simulink model "F18_Sim_animateFG4"  (R2014a)
settings: Solver=ode45  StartTime=0.0  StopTime=sim_time  RelTol=1e-3
values from neighbouring files (symbols this model uses):
  enableRT = 1    [F18_Animation_run3.m]    (also in f18full_DUopenloop_run1.m)
  h_ref = 0    [F18_Animation_run3.m]
  speedRT = 1    [F18_Animation_run3.m]
undefined symbols (not defined in the file or in its folder): Earth, WGS84
libraries: aerolibfltsims x4, aerolibanimutils x1, aerolibtransform2 x1
settings Model: Creator=Mishah  LastModifiedBy=changbc
settings DataIOCC: ExternalInput=[t, y, u]  LimitDataPoints=off  LoadExternalInput=on  SaveOutput=off  SignalLogging=off  SaveTime=off
settings OptimizationCC: ExpressionDepthLimit=2147483647
settings DebuggingCC: UnderspecifiedInitializationDetection=Classic  StateNameClashWarn=warning
settings GRTTargetCC: CombineOutputUpdateFcns=off  GRTInterface=on

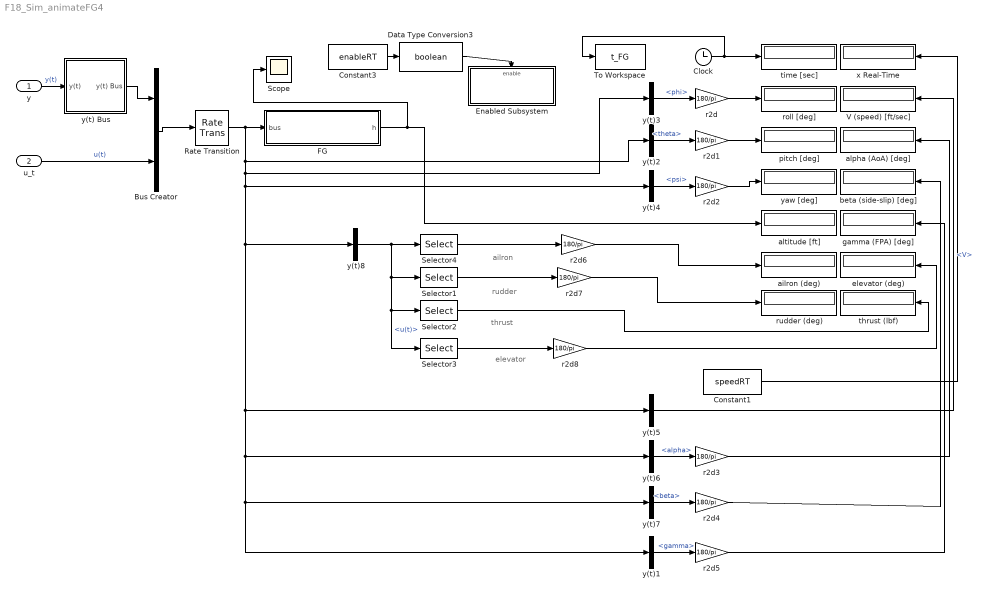
== system F18_Sim_animateFG4 ==
  note: ailron
  note: rudder
  note: thrust
  note: elevator
  y : Inport
  u_t : Inport  Port=2
  Bus Creator : BusCreator  Inputs=2
  Clock : Clock
  Constant1 : Constant  Value=speedRT
  Constant3 : Constant  Value=enableRT
  Data Type Conversion3 : DataTypeConversion  OutDataTypeStr=boolean
  Enabled Subsystem : Subsystem  TreatAsAtomicUnit=on
  FG : Subsystem
  Rate Transition : RateTransition
  Scope : Scope
      settings: YMin=-1000  YMax=12000
  Selector1 : Selector  InputPortWidth=4  Indices=2
  Selector2 : Selector  InputPortWidth=4  Indices=4
  Selector3 : Selector  InputPortWidth=4  Indices=3
  Selector4 : Selector  InputPortWidth=4
  To Workspace : ToWorkspace  VariableName=t_FG  SaveFormat=Structure  SampleTime=-1
  V (speed) [ft/sec] : Display
      settings: Format=bank
  ailron (deg) : Display
      settings: Format=bank
  alpha (AoA) [deg] : Display
      settings: Format=bank
  altitude [ft] : Display
      settings: Format=bank
  beta (side-slip) [deg] : Display
      settings: Format=bank
  elevator (deg) : Display
      settings: Format=bank
  gamma (FPA) [deg] : Display
      settings: Format=bank
  pitch [deg] : Display
      settings: Format=bank
  r2d{,1..8} (9 alike) : Gain  Gain=180/pi
  roll [deg] : Display
      settings: Format=bank
  rudder (deg) : Display
      settings: Format=bank
  thrust (lbf) : Display
      settings: Format=bank
  time [sec] : Display
      settings: Format=bank
  x Real-Time : Display
      settings: Format=bank
  y(t) Bus : Subsystem
  y(t)1 : BusSelector  OutputSignals=y(t) bus.uvwg.gamma
  y(t)2 : BusSelector  OutputSignals=y(t) bus.euler.theta
  y(t)3 : BusSelector  OutputSignals=y(t) bus.euler.phi
  y(t)4 : BusSelector  OutputSignals=y(t) bus.euler.psi
  y(t)5 : BusSelector  OutputSignals=y(t) bus.V;beta;alpha.V
  y(t)6 : BusSelector  OutputSignals=y(t) bus.V;beta;alpha.alpha
  y(t)7 : BusSelector  OutputSignals=y(t) bus.V;beta;alpha.beta
  y(t)8 : BusSelector  OutputSignals=u(t)
  yaw [deg] : Display
      settings: Format=bank
  wires:
  Constant3/1 -> Data Type Conversion3/1
  Rate Transition/1 -> y(t)7/1, y(t)1/1, y(t)6/1, y(t)5/1, y(t)8/1, y(t)4/1, y(t)3/1, y(t)2/1, FG/1(bus)
  y(t) Bus/1(y(t) Bus) -> Bus Creator/1
  u_t/1 -> Bus Creator/2  "u(t)"
  Clock/1 -> time [sec]/1, To Workspace/1
  Bus Creator/1 -> Rate Transition/1
  y(t)3/1 -> r2d/1  "<phi>"
  r2d/1 -> roll [deg]/1
  y(t)2/1 -> r2d1/1  "<theta>"
  r2d1/1 -> pitch [deg]/1
  y(t)4/1 -> r2d2/1  "<psi>"
  r2d2/1 -> yaw [deg]/1
  y(t)5/1 -> V (speed) [ft/sec]/1  "<V>"
  y(t)6/1 -> r2d3/1  "<alpha>"
  r2d3/1 -> alpha (AoA) [deg]/1
  y(t)7/1 -> r2d4/1  "<beta>"
  r2d4/1 -> beta (side-slip) [deg]/1
  y(t)1/1 -> r2d5/1  "<gamma>"
  r2d5/1 -> gamma (FPA) [deg]/1
  Data Type Conversion3/1 -> Enabled Subsystem/Enable
  Constant1/1 -> x Real-Time/1
  y/1 -> y(t) Bus/1(y(t))  "y(t)"
  FG/1(h) -> altitude [ft]/1, Scope/1
  y(t)8/1 -> Selector4/1, Selector1/1, Selector2/1, Selector3/1  "<u(t)>"
  Selector4/1 -> r2d6/1
  Selector1/1 -> r2d7/1
  Selector2/1 -> thrust (lbf)/1
  Selector3/1 -> r2d8/1
  r2d6/1 -> ailron (deg)/1
  r2d7/1 -> rudder (deg)/1
  r2d8/1 -> elevator (deg)/1

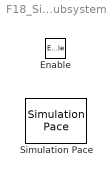
== system F18_Sim_animateFG4/Enabled Subsystem ==
  Enable : EnablePort
  Simulation Pace : aerolibanimutils/Simulation Pace  SimulationPace=1  SleepMode=MATLAB Thread  OutputPaceError=off  SampleTime=1/100
      settings: AttributesFormatString=%<SimulationPace> sec/sec

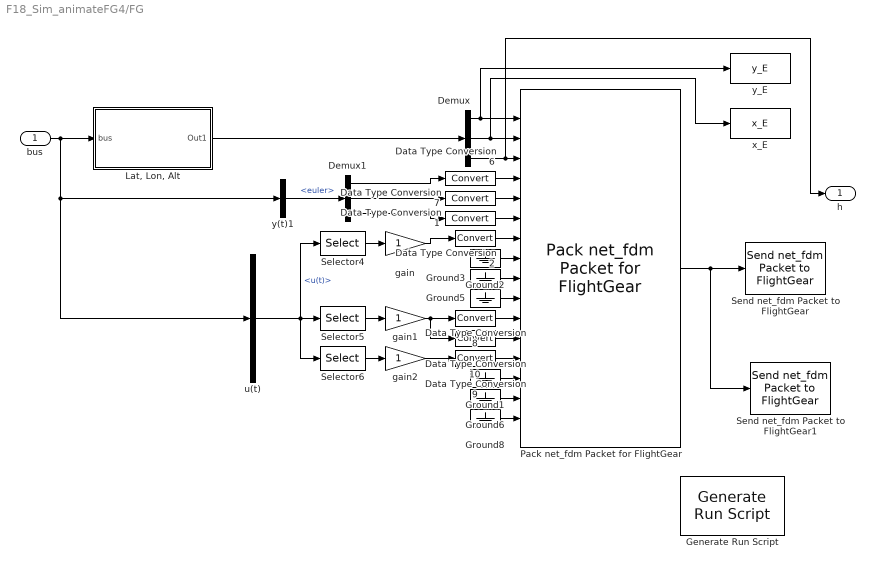
== system F18_Sim_animateFG4/FG ==
  bus : Inport
  Data Type Conversion{1..2,6..10} (7 alike) : DataTypeConversion
  Demux : Demux  Outputs=3
  Demux1 : Demux  Outputs=3
  Generate Run Script : aerolibfltsims/Generate Run Script  OutputFileName=runfg.bat  FlightGearBaseDirectory=C:\Program Files\FlightGear  GeometryModelName=ufo  DestinationPort=5502  OriginAddress=127.0.0.1  OriginPort=5505  LocalAddress=127.0.0.1  AirportId=REMOVE_THIS_LINE_FROM_SCRIPT  RunwayId=10L  InitialAltitude=100  InitialHeading=0  OffsetDistance=0  OffsetAzimuth=0  GenerateFile=off  Architecture=Default  dataFlow=Send
  Ground{1..3,5..6,8} (6 alike) : Ground
  "Lat, Lon, Alt" : Subsystem
  Pack net_fdm Packet for FlightGear : aerolibfltsims/Pack net_fdm Packet for FlightGear  FlightGearVersion=v2.12  ShowPositionAttitudeInputs=on  ShowVelocityAccelerationInputs=off  ShowControlSurfacePositionInputs=on  ShowEngineFuelInputs=off  ShowLandingGearInputs=off  ShowEnvironmentInputs=off  SampleTime=-1
  Selector4 : Selector  InputPortWidth=4  Indices=2
  Selector5 : Selector  InputPortWidth=4  Indices=3
  Selector6 : Selector  InputPortWidth=4  Indices=4
  Send net_fdm Packet to FlightGear : aerolibfltsims/Send net_fdm Packet to FlightGear  DestinationIpAddress=127.0.0.1  DestinationPort=5502  LocalIpPort=-1  varLen=off  SampleTime=-1
  Send net_fdm Packet to FlightGear1 : aerolibfltsims/Send net_fdm Packet to FlightGear  DestinationIpAddress=127.0.0.1  DestinationPort=5602  LocalIpPort=-1  varLen=off  SampleTime=-1
  gain : Gain
  gain1 : Gain
  gain2 : Gain
  u(t) : BusSelector  OutputSignals=u(t)
  x_E : ToWorkspace  VariableName=x_E  SaveFormat=Structure  SampleTime=-1
  y(t)1 : BusSelector  OutputSignals=y(t) bus.euler
  y_E : ToWorkspace  VariableName=y_E  SaveFormat=Structure  SampleTime=-1
  h : Outport
  wires:
  Ground2/1 -> Pack net_fdm Packet for FlightGear/8
  Ground8/1 -> Pack net_fdm Packet for FlightGear/16
  Ground6/1 -> Pack net_fdm Packet for FlightGear/15
  Data Type Conversion9/1 -> Pack net_fdm Packet for FlightGear/13
  Data Type Conversion10/1 -> Pack net_fdm Packet for FlightGear/12
  Data Type Conversion8/1 -> Pack net_fdm Packet for FlightGear/11
  Ground5/1 -> Pack net_fdm Packet for FlightGear/10
  Ground3/1 -> Pack net_fdm Packet for FlightGear/9
  y(t)1/1 -> Demux1/1  "<euler>"
  Data Type Conversion2/1 -> Pack net_fdm Packet for FlightGear/7
  Data Type Conversion1/1 -> Pack net_fdm Packet for FlightGear/6
  Data Type Conversion7/1 -> Pack net_fdm Packet for FlightGear/5
  Data Type Conversion6/1 -> Pack net_fdm Packet for FlightGear/4
  Ground1/1 -> Pack net_fdm Packet for FlightGear/14
  Demux1/3 -> Data Type Conversion1/1
  Demux1/2 -> Data Type Conversion7/1
  Demux1/1 -> Data Type Conversion6/1
  Demux/3 -> Pack net_fdm Packet for FlightGear/3, h/1
  Demux/2 -> Pack net_fdm Packet for FlightGear/2, x_E/1
  Demux/1 -> Pack net_fdm Packet for FlightGear/1, y_E/1
  Pack net_fdm Packet for FlightGear/1 -> Send net_fdm Packet to FlightGear1/1, Send net_fdm Packet to FlightGear/1
  "Lat, Lon, Alt"/1(Out1) -> Demux/1
  u(t)/1 -> Selector4/1, Selector5/1, Selector6/1  "<u(t)>"
  Selector4/1 -> gain/1
  Selector5/1 -> gain1/1
  Selector6/1 -> gain2/1
  gain1/1 -> Data Type Conversion8/1, Data Type Conversion10/1
  gain2/1 -> Data Type Conversion9/1
  gain/1 -> Data Type Conversion2/1
  bus/1 -> u(t)/1, y(t)1/1, "Lat, Lon, Alt"/1(bus)

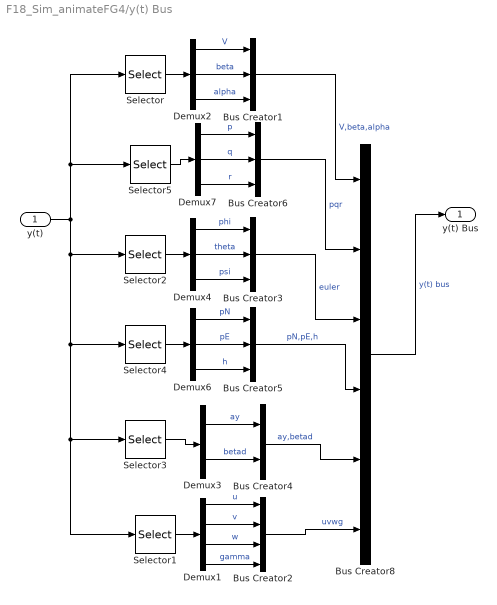
== system F18_Sim_animateFG4/y(t) Bus ==
  y(t) : Inport
  Bus Creator{1,3,5..6} (4 alike) : BusCreator  Inputs=3
  Bus Creator2 : BusCreator
  Bus Creator4 : BusCreator  Inputs=2
  Bus Creator8 : BusCreator  Inputs=6
  Demux1 : Demux
  Demux{2,4,6..7} (4 alike) : Demux  Outputs=3
  Demux3 : Demux  Outputs=2
  Selector : Selector  InputPortWidth=18  Indices=[1 2 3]
  Selector1 : Selector  InputPortWidth=18  Indices=[15 16 17 18]
  Selector2 : Selector  InputPortWidth=18  Indices=[7 8 9]
  Selector3 : Selector  InputPortWidth=18  Indices=[13 14]
  Selector4 : Selector  InputPortWidth=18  Indices=[10 11 12]
  Selector5 : Selector  InputPortWidth=18  Indices=[4 5 6]
  y(t) Bus : Outport
  wires:
  Bus Creator3/1 -> Bus Creator8/3  "euler"
  Bus Creator1/1 -> Bus Creator8/1  "V,beta,alpha"
  Demux7/3 -> Bus Creator6/3  "r"
  Selector5/1 -> Demux7/1
  Demux7/2 -> Bus Creator6/2  "q"
  Demux7/1 -> Bus Creator6/1  "p"
  Demux6/3 -> Bus Creator5/3  "h"
  Selector4/1 -> Demux6/1
  Demux6/2 -> Bus Creator5/2  "pE"
  Demux6/1 -> Bus Creator5/1  "pN"
  Demux4/3 -> Bus Creator3/3  "psi"
  Selector2/1 -> Demux4/1
  Demux4/2 -> Bus Creator3/2  "theta"
  Demux4/1 -> Bus Creator3/1  "phi"
  Selector/1 -> Demux2/1
  Demux2/3 -> Bus Creator1/3  "alpha"
  Demux2/2 -> Bus Creator1/2  "beta"
  Demux2/1 -> Bus Creator1/1  "V"
  y(t)/1 -> Selector2/1, Selector4/1, Selector1/1, Selector3/1, Selector/1, Selector5/1
  Bus Creator8/1 -> y(t) Bus/1  "y(t) bus"
  Bus Creator6/1 -> Bus Creator8/2  "pqr"
  Bus Creator5/1 -> Bus Creator8/4  "pN,pE,h"
  Demux1/3 -> Bus Creator2/3  "w"
  Selector1/1 -> Demux1/1
  Demux1/2 -> Bus Creator2/2  "v"
  Demux1/1 -> Bus Creator2/1  "u"
  Demux1/4 -> Bus Creator2/4  "gamma"
  Bus Creator2/1 -> Bus Creator8/6  "uvwg"
  Selector3/1 -> Demux3/1
  Demux3/1 -> Bus Creator4/1  "ay"
  Demux3/2 -> Bus Creator4/2  "betad"
  Bus Creator4/1 -> Bus Creator8/5  "ay,betad"

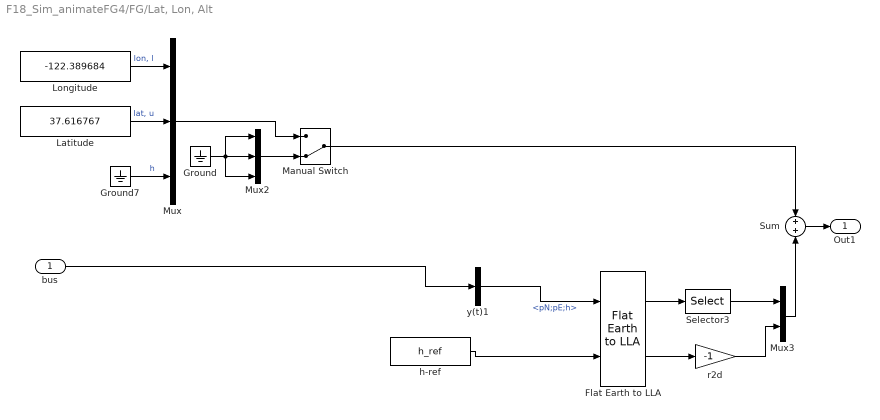
== system F18_Sim_animateFG4/FG/Lat, Lon, Alt ==
  bus : Inport
  Flat Earth to LLA : aerolibtransform2/Flat Earth to LLA  units=English  ptype=Earth (WGS84)  F=1/298.257223563  R=20925646.3255  LL0=[0 0]  psi=0
  Ground : Ground
  Ground7 : Ground
  Latitude : Constant  Value=37.616767
  Longitude : Constant  Value=-122.389684
  Manual Switch : ManualSwitch  CurrentSetting=0
  Mux : Mux  Inputs=3
  Mux2 : Mux  Inputs=3
  Mux3 : Mux  Inputs=2
  Selector3 : Selector  InputPortWidth=2  Indices=[2,1]
  Sum : Sum
  h-ref : Constant  Value=h_ref
  r2d : Gain  Gain=-1
  y(t)1 : BusSelector  OutputSignals=y(t) bus.pN;pE;h
  Out1 : Outport
  wires:
  Mux/1 -> Manual Switch/1
  Mux2/1 -> Manual Switch/2
  Ground7/1 -> Mux/3  "h"
  Latitude/1 -> Mux/2  "lat, u"
  Longitude/1 -> Mux/1  "lon, l"
  Flat Earth to LLA/1 -> Selector3/1
  Selector3/1 -> Mux3/1
  Flat Earth to LLA/2 -> r2d/1
  Ground/1 -> Mux2/1, Mux2/2, Mux2/3
  Manual Switch/1 -> Sum/1
  Mux3/1 -> Sum/2
  Sum/1 -> Out1/1
  h-ref/1 -> Flat Earth to LLA/2
  bus/1 -> y(t)1/1
  y(t)1/1 -> Flat Earth to LLA/1  "<pN;pE;h>"
  r2d/1 -> Mux3/2
